simulink subsystem "VehicleSimulationRef"  (R2024b)
settings: Solver=VariableStepAuto  StartTime=0.0  StopTime=10.0  RelTol=1e-3
undefined symbols (not defined in the file): damp, flightTrajectory, Ka_accel, Kd_rate, Ki_angle, Kp_angle, omega, resetFlag, SimIn, SimPar, trajLen
libraries: starslibAxisTransformations x6, simulink_extras x5, dspstat3 x3, vrlib x3, aerolibanimutils x2, dspnetwork x1, aerolibfltsims x1, simulink x1
(part 2 of 2)

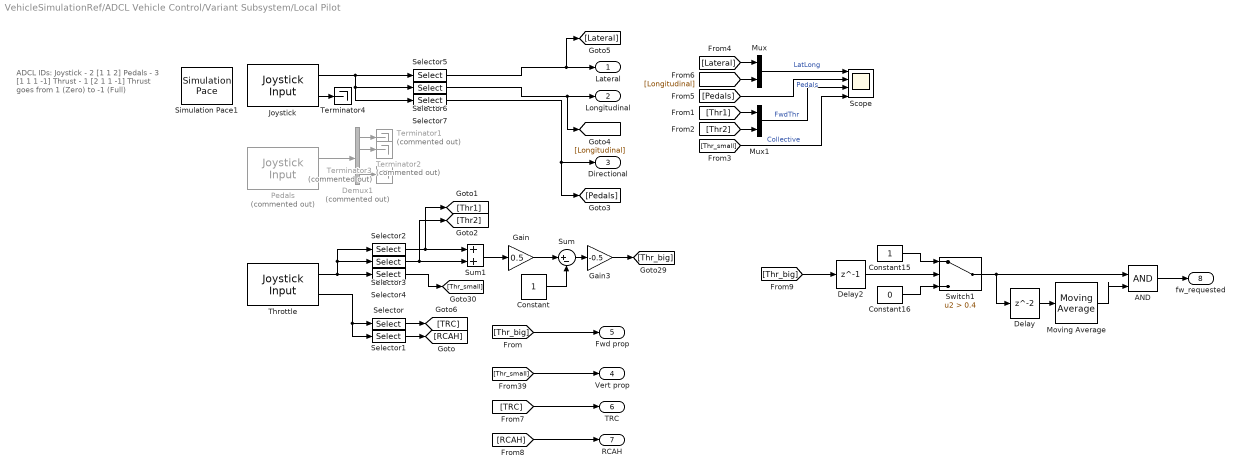
== system VehicleSimulationRef/ADCL Vehicle Control/Variant Subsystem/Local Pilot ==
  note: ADCL IDs:
      | Joystick - 2 [1 1 2]
      | Pedals - 3 [1 1 1 -1]
      | Thrust - 1 [2 1 1 -1]
      |
      | Thrust goes from 1 (Zero) to -1 (Full)
  AND : Logic  IconShape=distinctive  AllPortsSameDT=off  OutDataTypeStr=boolean
  Constant : Constant
  Constant15 : Constant
  Constant16 : Constant  Value=0
  Delay : Delay  InputProcessing=Columns as channels (frame based)  SampleTime=SimIn.Environment.Turbulence.dT
  Delay2 : Delay  DelayLength=1
  Demux1 : Demux  Commented=on  Outputs=[1 1 1 -1]
  Gain : Gain  Gain=0.5
  Gain3 : Gain  Gain=-0.5
  Joystick : vrlib/Joystick Input  joyid=2  adjustports=on  forcefeed=off
  Moving Average : dspstat3/Moving Average  Method=Sliding window  ForgettingFactorPort=off  SpecifyWindowLength=on  WindowLength=50  OverlapLength=49  AllowArbitraryInputLength=off  ForgettingFactor=0.9  SimulateUsing=Interpreted execution
  Mux : Mux  Inputs=2
  Mux1 : Mux  Inputs=2
  Pedals : vrlib/Joystick Input  Commented=on  joyid=3  adjustports=off  forcefeed=off
  Scope : Scope  NumInputPorts=4
  Selector : Selector  InputPortWidth=32  IndexOptions=Index vector (dialog)  Indices=24  OutputSizes=1
  Selector1 : Selector  InputPortWidth=32  IndexOptions=Index vector (dialog)  Indices=25  OutputSizes=1
  Selector2 : Selector  InputPortWidth=7  IndexOptions=Index vector (dialog)  Indices=3  OutputSizes=1
  Selector3 : Selector  InputPortWidth=7  IndexOptions=Index vector (dialog)  Indices=4  OutputSizes=1
  Selector4 : Selector  InputPortWidth=7  IndexOptions=Index vector (dialog)  Indices=5  OutputSizes=1
  Selector5 : Selector  InputPortWidth=4  IndexOptions=Index vector (dialog)  Indices=1  OutputSizes=1
  Selector6 : Selector  InputPortWidth=4  IndexOptions=Index vector (dialog)  Indices=2  OutputSizes=1
  Selector7 : Selector  InputPortWidth=4  IndexOptions=Index vector (dialog)  Indices=3  OutputSizes=1
  Simulation Pace1 : aerolibanimutils/Simulation Pace  SimulationPace=1  SleepMode=Auto  OutputPaceError=off  SampleTime=SimIn.Environment.Turbulence.dT
  Sum : Sum  Inputs=|+-
  Sum1 : Sum
  Switch1 : Switch  Criteria=u2 > Threshold  Threshold=0.4  SaturateOnIntegerOverflow=off  InputSameDT=off
  Terminator1 : Terminator  Commented=on
  Terminator2 : Terminator  Commented=on
  Terminator3 : Terminator  Commented=on
  Terminator4 : Terminator
  Throttle : vrlib/Joystick Input  joyid=1  adjustports=on  forcefeed=off
  Lateral : Outport
  Longitudinal : Outport  Port=2
  Directional : Outport  Port=3
  Vert prop : Outport  Port=4
  Fwd prop : Outport  Port=5
  TRC : Outport  Port=6
  RCAH : Outport  Port=7
  fw_requested : Outport  Port=8
  wires:
  [Thr_big] -> Delay2/1
  Constant16/1 -> Switch1/3
  Delay2/1 -> Switch1/2
  AND/1 -> fw_requested/1
  Constant15/1 -> Switch1/1
  Moving Average/1 -> AND/2
  Switch1/1 -> AND/1, Delay/1
  Delay/1 -> Moving Average/1
  Selector6/1 -> Longitudinal/1, [Longitudinal]
  Selector5/1 -> Lateral/1, [Lateral]
  Joystick/1 -> Selector5/1, Selector6/1, Selector7/1
  Selector1/1 -> [RCAH]
  [RCAH] -> RCAH/1
  [Thr_small] -> Vert prop/1
  [TRC] -> TRC/1
  Selector/1 -> [TRC]
  Throttle/2 -> Selector/1, Selector1/1
  [Thr_small] -> Scope/4  "Collective"
  Mux1/1 -> Scope/3  "FwdThr"
  [Pedals] -> Scope/2  "Pedals"
  Mux/1 -> Scope/1  "LatLong"
  [Thr2] -> Mux1/2
  [Thr1] -> Mux1/1
  [Lateral] -> Mux/1
  [Longitudinal] -> Mux/2
  Selector7/1 -> Directional/1, [Pedals]
  [Thr_big] -> Fwd prop/1
  Demux1/1 -> Terminator1/1
  Demux1/2 -> Terminator2/1
  Demux1/4 -> Terminator3/1
  Pedals/1 -> Demux1/1
  Gain3/1 -> [Thr_big]
  Constant/1 -> Sum/2
  Sum/1 -> Gain3/1
  Throttle/1 -> Selector4/1, Selector3/1, Selector2/1
  Sum1/1 -> Gain/1
  Selector2/1 -> [Thr1], Sum1/1
  Gain/1 -> Sum/1
  Selector3/1 -> [Thr2], Sum1/2
  Selector4/1 -> [Thr_small]
  Joystick/2 -> Terminator4/1

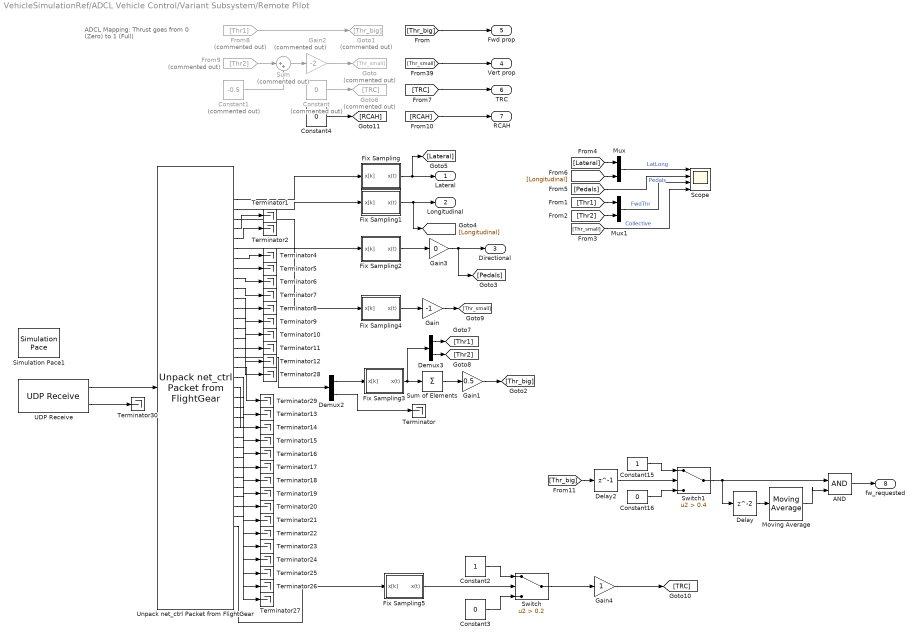
== system VehicleSimulationRef/ADCL Vehicle Control/Variant Subsystem/Remote Pilot ==
  note: ADCL Mapping:
      |
      | Thrust goes from 0 (Zero) to 1 (Full)
  AND : Logic  IconShape=distinctive  AllPortsSameDT=off  OutDataTypeStr=boolean
  Constant : Constant  Commented=on  Value=0
  Constant1 : Constant  Commented=on  Value=-0.5
  Constant15 : Constant
  Constant16 : Constant  Value=0
  Constant2 : Constant
  Constant3 : Constant  Value=0
  Constant4 : Constant  Value=0
  Delay : Delay  InputProcessing=Columns as channels (frame based)  SampleTime=SimIn.Environment.Turbulence.dT
  Delay2 : Delay  DelayLength=1
  Demux2 : Demux  Outputs=[2 2]
  Demux3 : Demux  Outputs=2
  Fix Sampling : Subsystem
  Fix Sampling1 : Subsystem
  Fix Sampling2 : Subsystem
  Fix Sampling3 : Subsystem
  Fix Sampling4 : Subsystem
  Fix Sampling5 : Subsystem
  From8 : From  Commented=on  GotoTag=Thr1
  From9 : From  Commented=on  GotoTag=Thr2
  Gain : Gain  Gain=-1
  Gain1 : Gain  Gain=0.5
  Gain2 : Gain  Commented=on  Gain=-2
  Gain3 : Gain  Gain=0
  Gain4 : Gain
  Goto : Goto  Commented=on  GotoTag=Thr_small
  Goto1 : Goto  Commented=on  GotoTag=Thr_big
  Goto6 : Goto  Commented=on  GotoTag=TRC
  Moving Average : dspstat3/Moving Average  Method=Sliding window  ForgettingFactorPort=off  SpecifyWindowLength=on  WindowLength=50  OverlapLength=49  AllowArbitraryInputLength=off  ForgettingFactor=0.9  SimulateUsing=Interpreted execution
  Mux : Mux  Inputs=2
  Mux1 : Mux  Inputs=2
  Scope : Scope  NumInputPorts=4
  Simulation Pace1 : aerolibanimutils/Simulation Pace  SimulationPace=1  SleepMode=Auto  OutputPaceError=off  SampleTime=SimIn.Environment.Turbulence.dT
  Sum : Sum  Commented=on  Inputs=|++
  Sum of Elements : Sum  Inputs=+
  Switch : Switch  Criteria=u2 > Threshold  Threshold=0.2  SaturateOnIntegerOverflow=off  InputSameDT=off
  Switch1 : Switch  Criteria=u2 > Threshold  Threshold=0.4  SaturateOnIntegerOverflow=off  InputSameDT=off
  Terminator{,1..2,4..30} (30 alike) : Terminator
  UDP Receive : dspnetwork/UDP Receive  localURL='0.0.0.0'  localPort=SimIn.simPortOutput  remoteURL=SimIn.simAddress  remotePort=-1  recvBufferSize=8192  dims=744  signalDatatype=uint8  isComplex=off  isVarSize=off  showBlockingTime=off  blockingTime=0  sampletime=-1  blockPlatform=[]
      settings: LibrarySourceBlock=dspsrcs4/UDP Receive
  Unpack net_ctrl Packet from FlightGear : aerolibfltsims/Unpack net_ctrl Packet from FlightGear  FlightGearVersion=v2019.1  ShowControlSurfacePositionOutputs=on  ShowEngineFuelOutputs=on  ShowLandingGearOutputs=on  ShowAvionicOutputs=off  ShowEnvironmentOutputs=off  SampleTime=-1  packetVersion=27
  Lateral : Outport
  Longitudinal : Outport  Port=2
  Directional : Outport  Port=3
  Vert prop : Outport  Port=4
  Fwd prop : Outport  Port=5
  TRC : Outport  Port=6
  RCAH : Outport  Port=7
  fw_requested : Outport  Port=8
  wires:
  Delay2/1 -> Switch1/2
  Constant16/1 -> Switch1/3
  Moving Average/1 -> AND/2
  Constant15/1 -> Switch1/1
  Switch1/1 -> AND/1, Delay/1
  [Thr_big] -> Delay2/1
  Delay/1 -> Moving Average/1
  AND/1 -> fw_requested/1
  Gain4/1 -> [TRC]
  Constant4/1 -> [RCAH]
  [RCAH] -> RCAH/1
  [TRC] -> TRC/1
  Switch/1 -> Gain4/1
  Constant3/1 -> Switch/3
  Constant2/1 -> Switch/1
  Unpack net_ctrl Packet from FlightGear/34 -> Fix Sampling5/1(x[k])
  Fix Sampling5/1(x(t)) -> Switch/2
  Gain3/1 -> [Pedals], Directional/1
  Gain/1 -> [Thr_small]
  Unpack net_ctrl Packet from FlightGear/6 -> Fix Sampling4/1(x[k])
  Fix Sampling4/1(x(t)) -> Gain/1
  Gain2/1 -> Goto/1
  Sum/1 -> Gain2/1
  From9/1 -> Sum/1
  Constant1/1 -> Sum/2
  From8/1 -> Goto1/1
  Fix Sampling3/1(x(t)) -> Sum of Elements/1, Demux3/1
  Fix Sampling2/1(x(t)) -> Gain3/1
  Fix Sampling1/1(x(t)) -> [Longitudinal], Longitudinal/1
  Fix Sampling/1(x(t)) -> [Lateral], Lateral/1
  UDP Receive/1 -> Unpack net_ctrl Packet from FlightGear/1
  UDP Receive/2 -> Terminator30/1
  Unpack net_ctrl Packet from FlightGear/18 -> Terminator29/1
  Unpack net_ctrl Packet from FlightGear/16 -> Terminator28/1
  Unpack net_ctrl Packet from FlightGear/33 -> Terminator27/1
  Unpack net_ctrl Packet from FlightGear/32 -> Terminator26/1
  Unpack net_ctrl Packet from FlightGear/31 -> Terminator25/1
  Unpack net_ctrl Packet from FlightGear/30 -> Terminator24/1
  Unpack net_ctrl Packet from FlightGear/29 -> Terminator23/1
  Unpack net_ctrl Packet from FlightGear/28 -> Terminator22/1
  Unpack net_ctrl Packet from FlightGear/27 -> Terminator21/1
  Unpack net_ctrl Packet from FlightGear/26 -> Terminator20/1
  Unpack net_ctrl Packet from FlightGear/25 -> Terminator19/1
  Unpack net_ctrl Packet from FlightGear/24 -> Terminator18/1
  Unpack net_ctrl Packet from FlightGear/23 -> Terminator17/1
  Unpack net_ctrl Packet from FlightGear/22 -> Terminator16/1
  Unpack net_ctrl Packet from FlightGear/21 -> Terminator15/1
  Unpack net_ctrl Packet from FlightGear/20 -> Terminator14/1
  Unpack net_ctrl Packet from FlightGear/19 -> Terminator13/1
  Unpack net_ctrl Packet from FlightGear/15 -> Terminator12/1
  Unpack net_ctrl Packet from FlightGear/14 -> Terminator11/1
  Unpack net_ctrl Packet from FlightGear/13 -> Terminator10/1
  Unpack net_ctrl Packet from FlightGear/12 -> Terminator9/1
  Unpack net_ctrl Packet from FlightGear/11 -> Terminator8/1
  Unpack net_ctrl Packet from FlightGear/10 -> Terminator7/1
  Unpack net_ctrl Packet from FlightGear/9 -> Terminator6/1
  Unpack net_ctrl Packet from FlightGear/8 -> Terminator5/1
  Unpack net_ctrl Packet from FlightGear/7 -> Terminator4/1
  Unpack net_ctrl Packet from FlightGear/5 -> Terminator2/1
  Unpack net_ctrl Packet from FlightGear/4 -> Terminator1/1
  Constant/1 -> Goto6/1
  Demux2/2 -> Terminator/1
  Gain1/1 -> [Thr_big]
  Demux3/2 -> [Thr2]
  Demux3/1 -> [Thr1]
  Unpack net_ctrl Packet from FlightGear/1 -> Fix Sampling/1(x[k])
  Unpack net_ctrl Packet from FlightGear/2 -> Fix Sampling1/1(x[k])
  [Thr_big] -> Fwd prop/1
  [Thr_small] -> Vert prop/1
  Unpack net_ctrl Packet from FlightGear/3 -> Fix Sampling2/1(x[k])
  [Longitudinal] -> Mux/2
  [Lateral] -> Mux/1
  [Thr1] -> Mux1/1
  [Thr2] -> Mux1/2
  Mux/1 -> Scope/1  "LatLong"
  [Pedals] -> Scope/2  "Pedals"
  Mux1/1 -> Scope/3  "FwdThr"
  [Thr_small] -> Scope/4  "Collective"
  Unpack net_ctrl Packet from FlightGear/17 -> Demux2/1
  Demux2/1 -> Fix Sampling3/1(x[k])
  Sum of Elements/1 -> Gain1/1

== system VehicleSimulationRef/ADCL Vehicle Control/Mapping To Output/Eng Dynamics Compensation/Default ==
  Eng_Des : Inport
  Eng_Cmd : Outport
  wires:
  Eng_Des/1 -> Eng_Cmd/1

== system VehicleSimulationRef/ADCL Vehicle Control/Mapping To Output/Eng Dynamics Compensation/First Order ==
  note: “Cancel” the lag from the First Order dynamics by commanding a value that anticipates the needed deflection rate. This formula “inverts” the first-order lag.
  Eng_Des : Inport
  Derivative : Derivative
  Sum : Sum  Inputs=|++
  tau : Gain  Gain=1 ./ (2 * pi * SimPar.Engine.BW)
  Eng_Cmd : Outport
  wires:
  tau/1 -> Sum/2
  Sum/1 -> Eng_Cmd/1
  Derivative/1 -> tau/1
  Eng_Des/1 -> Derivative/1, Sum/1

== system VehicleSimulationRef/ADCL Vehicle Control/Mapping To Output/Surf Dynamics Compensation/Default ==
  Surf_Des : Inport
  Surf_Cmd : Outport
  wires:
  Surf_Des/1 -> Surf_Cmd/1

== system VehicleSimulationRef/ADCL Vehicle Control/Mapping To Output/Surf Dynamics Compensation/First Order ==
  note: “Cancel” the lag from the First Order dynamics by commanding a value that anticipates the needed deflection rate. This formula “inverts” the first-order lag.
  Surf_Des : Inport
  Derivative : Derivative
  Sum : Sum  Inputs=|++
  tau : Gain  Gain=1 ./ (2 * pi * SimPar.Actuator.BW)
  Surf_Cmd : Outport
  wires:
  tau/1 -> Sum/2
  Surf_Des/1 -> Sum/1, Derivative/1
  Derivative/1 -> tau/1
  Sum/1 -> Surf_Cmd/1

== system VehicleSimulationRef/ADCL Vehicle Control/Pilot Command Filtering/Translational Rate Command (TRC)/Linear controller ==
  ref : Inport
  ref_dot : Inport  Port=2
  x_dot : Inport  Port=3
  notTRC : Inport  Port=4
  Gain : Gain  Gain=Kp
  Gain1 : Gain  Gain=Ki
  Gain2 : Gain  Gain=Ka
  Integrator : Integrator  ExternalReset=level
  Sum : Sum  Inputs=|+-
  Sum1 : Sum  Inputs=+++
  req : Outport
  wires:
  notTRC/1 -> Integrator/2
  Gain2/1 -> Sum1/1
  ref_dot/1 -> Gain2/1
  Integrator/1 -> Sum1/3
  Gain/1 -> Sum1/2
  Sum1/1 -> req/1
  Gain1/1 -> Integrator/1
  Sum/1 -> Gain/1, Gain1/1
  x_dot/1 -> Sum/2
  ref/1 -> Sum/1

== system VehicleSimulationRef/ADCL Vehicle Control/Pilot Command Filtering/Translational Rate Command (TRC)/Reference model ==
  xy_dot_comm : Inport
  notTRC : Inport  Port=2
  xy_dot_0 : Inport  Port=3
  1/Tv : Gain  Gain=1/Tv
  Constant1 : Constant  Value=0
  Integrator : Integrator  ExternalReset=level  InitialConditionSource=external
  Sum : Sum  Inputs=|+-
  Switch : Switch  Criteria=u2 ~= 0  SaturateOnIntegerOverflow=off  InputSameDT=off
  ref : Outport
  ref_dot : Outport  Port=2
  wires:
  1/Tv/1 -> Switch/3
  Constant1/1 -> Switch/1
  xy_dot_0/1 -> Integrator/3
  notTRC/1 -> Integrator/2, Switch/2
  Sum/1 -> 1/Tv/1
  xy_dot_comm/1 -> Sum/1
  Switch/1 -> Integrator/1, ref_dot/1
  Integrator/1 -> Sum/2, ref/1

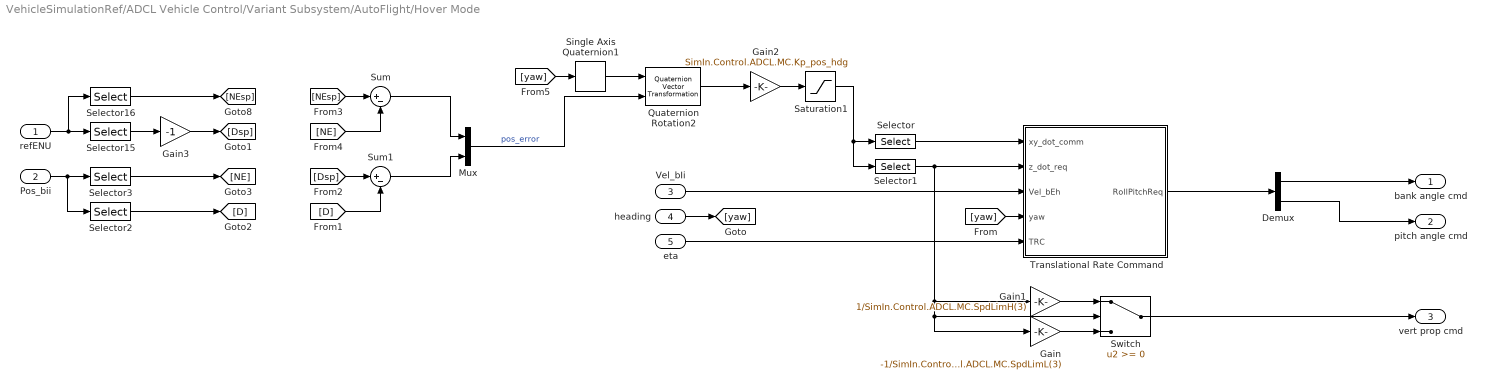
== system VehicleSimulationRef/ADCL Vehicle Control/Variant Subsystem/AutoFlight/Hover Mode ==
  refENU : Inport
  Pos_bii : Inport  Port=2
  Vel_bIi : Inport  Port=3
  heading : Inport  Port=4
  eta : Inport  Port=5
  Demux : Demux  Outputs=2
  Gain : Gain  Gain=-1/SimIn.Control.ADCL.MC.SpdLimL(3)
  Gain1 : Gain  Gain=1/SimIn.Control.ADCL.MC.SpdLimH(3)
  Gain2 : Gain  Gain=SimIn.Control.ADCL.MC.Kp_pos_hdg
  Gain3 : Gain  Gain=-1
  Mux : Mux  Inputs=2
  Quaternion Rotation2 : starslibAxisTransformations/Quaternion Vector Transformation  n=0
  Saturation1 : Saturate  UpperLimit=SimIn.Control.ADCL.MC.SpdLimH  LowerLimit=SimIn.Control.ADCL.MC.SpdLimL
  Selector : Selector  InputPortWidth=3  IndexOptions=Index vector (dialog)  Indices=[1 2]  OutputSizes=1
  Selector1 : Selector  InputPortWidth=3  IndexOptions=Index vector (dialog)  Indices=3  OutputSizes=1
  Selector15 : Selector  InputPortWidth=3  IndexOptions=Index vector (dialog)  Indices=3  OutputSizes=1
  Selector16 : Selector  InputPortWidth=3  IndexOptions=Index vector (dialog)  Indices=[2 1]  OutputSizes=1
  Selector2 : Selector  InputPortWidth=3  IndexOptions=Index vector (dialog)  Indices=3  OutputSizes=1
  Selector3 : Selector  InputPortWidth=3  IndexOptions=Index vector (dialog)  Indices=[1 2]  OutputSizes=1
  Single Axis Quaternion1 : starslibAxisTransformations/Single Axis Quaternion  RotAxis=z  n=0
  Sum : Sum  Inputs=|+-
  Sum1 : Sum  Inputs=|+-
  Switch : Switch  SaturateOnIntegerOverflow=off  InputSameDT=off
  Translational Rate Command : Subsystem
  bank angle cmd : Outport
  pitch angle cmd : Outport  Port=2
  vert prop cmd : Outport  Port=3
  wires:
  refENU/1 -> Selector16/1, Selector15/1
  Pos_bii/1 -> Selector2/1, Selector3/1
  Selector15/1 -> Gain3/1
  Selector16/1 -> [NEsp]
  Gain3/1 -> [Dsp]
  Selector3/1 -> [NE]
  Selector2/1 -> [D]
  Sum/1 -> Mux/1
  Sum1/1 -> Mux/2
  [D] -> Sum1/2
  [Dsp] -> Sum1/1
  [NEsp] -> Sum/1
  [NE] -> Sum/2
  Mux/1 -> Quaternion Rotation2/2  "pos_error"
  Saturation1/1 -> Selector/1, Selector1/1
  Gain2/1 -> Saturation1/1
  Quaternion Rotation2/1 -> Gain2/1
  Selector1/1 -> Translational Rate Command/2(z_dot_req), Switch/2, Gain/1, Gain1/1
  Selector/1 -> Translational Rate Command/1(xy_dot_comm)
  [yaw] -> Translational Rate Command/4(yaw)
  Single Axis Quaternion1/1 -> Quaternion Rotation2/1
  [yaw] -> Single Axis Quaternion1/1
  Gain1/1 -> Switch/1
  Gain/1 -> Switch/3
  heading/1 -> [yaw]
  Demux/2 -> pitch angle cmd/1
  Vel_bIi/1 -> Translational Rate Command/3(Vel_bEh)
  Translational Rate Command/1(RollPitchReq) -> Demux/1
  Switch/1 -> vert prop cmd/1
  eta/1 -> Translational Rate Command/5(TRC)
  Demux/1 -> bank angle cmd/1

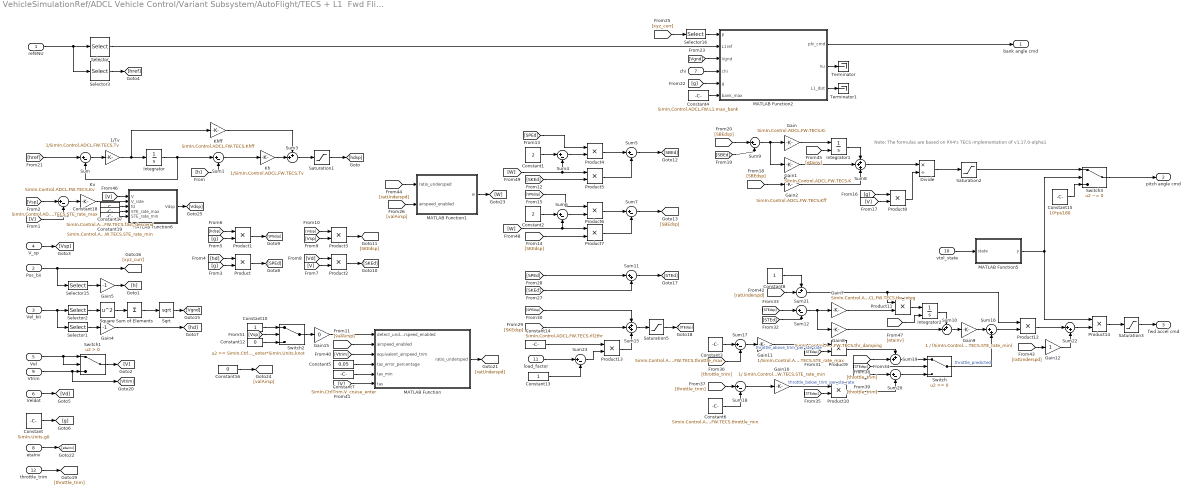
== system VehicleSimulationRef/ADCL Vehicle Control/Variant Subsystem/AutoFlight/TECS + L1  Fwd Flight ==
  note: Note: The formulas are based on PX4's TECS implementation of v1.17.0-alpha1
  refENU : Inport
  Pos_bii : Inport  Port=2
  Vel_bIi : Inport  Port=3
  V_sp : Inport  Port=4
  Vel : Inport  Port=5
  Veldot : Inport  Port=6
  chi : Inport  Port=7
  etaInv : Inport  Port=8
  Vtrim : Inport  Port=9
  vtol_state : Inport  Port=10
  load_factor : Inport  Port=11
  throttle_trim : Inport  Port=12
  1/Tv : Gain  Gain=1/SimIn.Control.ADCL.FW.TECS.Tv
  Constant : Constant  Value=SimIn.Units.g0
  Constant1 : Constant  Value=2
  Constant10 : Constant
  Constant12 : Constant  Value=0
  Constant13 : Constant
  Constant14 : Constant  Value=SimIn.Control.ADCL.FW.TECS.rll2thr
  Constant15 : Constant  Value=10*pi/180
  Constant16 : Constant  Value=0
  Constant17 : Constant  Value=SimIn.Control.ADCL.FW.TECS.fast_descend
  Constant18 : Constant  Value=SimIn.Control.ADCL.FW.TECS.STE_rate_max
  Constant19 : Constant  Value=SimIn.Control.ADCL.FW.TECS.STE_rate_min
  Constant2 : Constant  Value=2
  Constant3 : Constant  Value=SimIn.Control.ADCL.FW.TECS.throttle_max
  Constant4 : Constant  Value=SimIn.Control.ADCL.FW.L1.max_bank
  Constant5 : Constant  Value=0.05
  Constant6 : Constant  Value=SimIn.Control.ADCL.FW.TECS.throttle_min
  Constant7 : Constant  Value=SimIn.CtrlTrim.V_cruise_enter
  Constant8 : Constant
  Divide : Product  Inputs=*/
  Gain : Gain  Gain=SimIn.Control.ADCL.FW.TECS.Ki
  Gain1 : Gain  Gain=SimIn.Control.ADCL.FW.TECS.K
  Gain10 : Gain  Gain=1/ SimIn.Control.ADCL.FW.TECS.STE_rate_min
  Gain11 : Gain  Gain=1/SimIn.Control.ADCL.FW.TECS.STE_rate_max
  Gain12 : Gain
  Gain15 : Gain  Gain=0
  Gain2 : Gain  Gain=SimIn.Control.ADCL.FW.TECS.Kff
  Gain4 : Gain  Gain=-1
  Gain5 : Gain  Gain=-1
  Gain7 : Gain  Gain=SimIn.Control.ADCL.FW.TECS.thr_integ
  Gain8 : Gain  Gain=SimIn.Control.ADCL.FW.TECS.thr_damping
  Gain9 : Gain  Gain=1 / (SimIn.Control.ADCL.FW.TECS.STE_rate_max - SimIn.Control.ADCL.FW.TECS.STE_rate_min)
  Integrator : Integrator  InitialCondition=-SimIn.EOM.Pos_bii(3)
  Integrator1 : Integrator  ExternalReset=rising
  Integrator2 : Integrator  ExternalReset=rising
  Kh : Gain  Gain=1/SimIn.Control.ADCL.FW.TECS.Tv
  Khff : Gain  Gain=SimIn.Control.ADCL.FW.TECS.Khff
  Kv : Gain  Gain=SimIn.Control.ADCL.FW.TECS.Kv
  MATLAB Function : MATLAB Function  TreatAsAtomicUnit=on
  MATLAB Function1 : MATLAB Function  TreatAsAtomicUnit=on
  MATLAB Function2 : MATLAB Function  TreatAsAtomicUnit=on
  MATLAB Function5 : MATLAB Function  TreatAsAtomicUnit=on
  MATLAB Function6 : MATLAB Function  TreatAsAtomicUnit=on
  Product{,1..14} (15 alike) : Product
  Saturation1 : Saturate  UpperLimit=SimIn.Control.ADCL.FW.TECS.climb_rate  LowerLimit=-SimIn.Control.ADCL.FW.TECS.max_sink_rate
  Saturation2 : Saturate  UpperLimit=SimIn.Control.ADCL.FW.TECS.max_pitch  LowerLimit=SimIn.Control.ADCL.FW.TECS.min_pitch
  Saturation3 : Saturate  UpperLimit=SimIn.Control.ADCL.FW.TECS.throttle_max  LowerLimit=SimIn.Control.ADCL.FW.TECS.throttle_min
  Saturation5 : Saturate  UpperLimit=SimIn.Control.ADCL.FW.TECS.STE_rate_max  LowerLimit=SimIn.Control.ADCL.FW.TECS.STE_rate_min
  Selector : Selector  InputPortWidth=3  IndexOptions=Index vector (dialog)  Indices=[2 1]  OutputSizes=1
  Selector1 : Selector  InputPortWidth=3  IndexOptions=Index vector (dialog)  Indices=3  OutputSizes=1
  Selector15 : Selector  InputPortWidth=3  IndexOptions=Index vector (dialog)  Indices=3  OutputSizes=1
  Selector16 : Selector  InputPortWidth=3  IndexOptions=Index vector (dialog)  Indices=[1 2]  OutputSizes=1
  Selector2 : Selector  InputPortWidth=3  IndexOptions=Index vector (dialog)  Indices=[1 2]  OutputSizes=1
  Selector3 : Selector  InputPortWidth=3  IndexOptions=Index vector (dialog)  Indices=3  OutputSizes=1
  Sqrt : Sqrt
  Square : Math  Operator=square
  Sum{,1..2,4..7,9,12,17..18,20,23} (13 alike) : Sum  Inputs=|+-
  Sum of Elements : Sum  Inputs=+
  Sum10 : Sum  Inputs=++|
  Sum11 : Sum  Inputs=|++
  Sum15 : Sum  Inputs=+++
  Sum16 : Sum  Inputs=|++
  Sum19 : Sum  Inputs=++|
  Sum21 : Sum  Inputs=+-|
  Sum22 : Sum  Inputs=|++
  Sum3 : Sum  Inputs=++|
  Sum8 : Sum  Inputs=+++
  Switch : Switch  SaturateOnIntegerOverflow=off  InputSameDT=off
  Switch1 : Switch  Criteria=u2 > Threshold  SaturateOnIntegerOverflow=off  InputSameDT=off
  Switch2 : Switch  Threshold=SimIn.CtrlTrim.V_cruise_enter*SimIn.Units.knot  SaturateOnIntegerOverflow=off  InputSameDT=off
  Switch3 : Switch  Criteria=u2 ~= 0  SaturateOnIntegerOverflow=off  InputSameDT=off
  Terminator : Terminator
  Terminator1 : Terminator
  bank angle cmd : Outport
  pitch angle cmd : Outport  Port=2
  fwd accel cmd : Outport  Port=3
  wires:
  Selector3/1 -> [href]
  Selector/1 -> MATLAB Function2/2(L1ref)
  refENU/1 -> Selector/1, Selector3/1
  MATLAB Function6/1(Vdsp) -> [Vdsp]
  Constant18/1 -> MATLAB Function6/4(STE_rate_max)
  Constant19/1 -> MATLAB Function6/5(STE_rate_min)
  Constant17/1 -> MATLAB Function6/3(fd)
  [V] -> MATLAB Function6/1(V)
  Constant16/1 -> [valAirsp]
  Selector16/1 -> MATLAB Function2/1(p)
  MATLAB Function5/1(y) -> Switch3/2, Product14/1
  throttle_trim/1 -> [throttle_trim]
  vtol_state/1 -> MATLAB Function5/1(state)
  Switch3/1 -> pitch angle cmd/1
  Product14/1 -> Saturation3/1
  Constant15/1 -> Switch3/3
  Product12/1 -> Sum22/1
  Sum16/1 -> Product12/2
  MATLAB Function2/1(phi_cmd) -> bank angle cmd/1
  Saturation2/1 -> Switch3/1
  Saturation3/1 -> fwd accel cmd/1
  Gain15/1 -> MATLAB Function/1(detect_underspeed_enabled)
  Saturation5/1 -> [STEdsp]
  Product13/1 -> Sum15/3
  Constant14/1 -> Product13/1
  Sum23/1 -> Product13/2
  Constant13/1 -> Sum23/2
  load_factor/1 -> Sum23/1
  [W] -> Product5/1, Sum4/2
  MATLAB Function1/1(w) -> [W]
  [etainv] -> Integrator2/2
  [Vsp] -> Switch2/2
  etaInv/1 -> [etainv]
  Switch2/1 -> Gain15/1
  Constant12/1 -> Switch2/3
  Constant10/1 -> Switch2/1
  [valAirsp] -> MATLAB Function/2(airspeed_enabled)
  [valAirsp] -> MATLAB Function1/2(airspeed_enabled)
  [ratUnderspd] -> MATLAB Function1/1(ratio_undersped)
  Gain12/1 -> Sum22/2
  Sum22/1 -> Product14/2
  [ratUnderspd] -> Gain12/1
  Gain8/1 -> Sum10/2
  Sum21/1 -> Product11/1, Product12/1
  Gain7/1 -> Product11/2
  Product11/1 -> Integrator2/1
  Sum10/1 -> Gain9/1
  [ratUnderspd] -> Sum21/2
  Constant8/1 -> Sum21/1
  MATLAB Function/1(ratio_undersped) -> [ratUnderspd]
  Constant7/1 -> MATLAB Function/5(tas_min)
  Constant5/1 -> MATLAB Function/4(tas_error_percentage)
  [V] -> MATLAB Function/6(tas)
  [Vtrim] -> MATLAB Function/3(equivalent_airspeed_trim)
  Vtrim/1 -> Switch1/3, [Vtrim]
  Vel/1 -> Switch1/1, Switch1/2
  Switch1/1 -> [V]
  Gain11/1 -> Product9/1  "throttle_above_trim_per_ste_rate"
  Gain10/1 -> Product10/1  "throttle_below_trim_per_ste_rate"
  Product10/1 -> Sum20/2
  [throttle_trim] -> Sum20/1
  Sum20/1 -> Switch/3
  Sum19/1 -> Switch/1
  [throttle_trim] -> Sum19/2
  [throttle_trim] -> Sum18/1
  [throttle_trim] -> Sum17/2
  Constant6/1 -> Sum18/2
  [STEdsp] -> Product10/2
  Sum18/1 -> Gain10/1
  Sum17/1 -> Gain11/1
  [STEdsp] -> Product9/2
  Constant3/1 -> Sum17/1
  Gain9/1 -> Sum16/1
  Switch/1 -> Sum16/2  "throttle_predicted"
  Product9/1 -> Sum19/1
  [STEdsp] -> Switch/2
  Integrator2/1 -> Sum10/1
  Sum12/1 -> Gain8/1, Gain7/1
  [STEdsp] -> Sum12/1
  [STEd] -> Sum12/2
  [SKEdsp] -> Sum15/2
  [SPEdsp] -> Sum15/1
  [SKEd] -> Sum11/2
  [SPEd] -> Sum11/1
  Sum15/1 -> Saturation5/1
  Sum11/1 -> [STEd]
  [etainv] -> Integrator1/2
  [xyz_curr] -> Selector16/1
  Pos_bii/1 -> Selector15/1, [xyz_curr]
  [Vgnd] -> MATLAB Function2/3(Vgnd)
  Gain5/1 -> [h]
  Selector15/1 -> Gain5/1
  Gain4/1 -> [hd]
  Selector1/1 -> Gain4/1
  [href] -> Sum/1
  MATLAB Function2/3(L1_dist) -> Terminator1/1
  MATLAB Function2/2(nu) -> Terminator/1
  Sqrt/1 -> [Vgnd]
  Square/1 -> Sum of Elements/1
  Sum of Elements/1 -> Sqrt/1
  Selector2/1 -> Square/1
  Vel_bIi/1 -> Selector1/1, Selector2/1
  Khff/1 -> Sum3/1
  Kh/1 -> Sum3/2
  Constant4/1 -> MATLAB Function2/6(bank_max)
  [g] -> MATLAB Function2/5(g)
  chi/1 -> MATLAB Function2/4(chi)
  [SBEd] -> Sum9/2
  [SBEdsp] -> Sum9/1
  Sum9/1 -> Gain/1, Gain1/1
  Sum8/1 -> Divide/1
  Gain2/1 -> Sum8/3
  [SBEdsp] -> Gain2/1
  Integrator1/1 -> Sum8/1
  Gain1/1 -> Sum8/2
  Gain/1 -> Integrator1/1
  Divide/1 -> Saturation2/1
  Product8/1 -> Divide/2
  [g] -> Product8/1
  [V] -> Product8/2
  Sum5/1 -> [SBEd]
  Sum7/1 -> [SBEdsp]
  Constant2/1 -> Sum6/1
  Sum6/1 -> Product6/2
  Product6/1 -> Sum7/1
  Product7/1 -> Sum7/2
  [SPEdsp] -> Product6/1
  [SKEdsp] -> Product7/2
  [SKEd] -> Product5/2
  [SPEd] -> Product4/1
  Product5/1 -> Sum5/2
  Product4/1 -> Sum5/1
  Sum4/1 -> Product4/2
  [W] -> Product7/1, Sum6/2
  Constant1/1 -> Sum4/1
  [Vd] -> Product2/1
  [V] -> Product2/2
  Product2/1 -> [SKEd]
  Product3/1 -> [SKEdsp]
  [Vsp] -> Product3/2
  [Vdsp] -> Product3/1
  [hdsp] -> Product1/1
  [g] -> Product1/2
  Product1/1 -> [SPEdsp]
  Product/1 -> [SPEd]
  [g] -> Product/2
  [hd] -> Product/1
  Constant/1 -> [g]
  Saturation1/1 -> [hdsp]
  [Vsp] -> Sum2/1
  Veldot/1 -> [Vd]
  [V] -> Sum2/2
  Kv/1 -> MATLAB Function6/2(V_rate)
  [h] -> Sum1/2
  Sum3/1 -> Saturation1/1
  Sum1/1 -> Kh/1
  Sum2/1 -> Kv/1
  V_sp/1 -> [Vsp]
  1/Tv/1 -> Integrator/1, Khff/1
  Sum/1 -> 1/Tv/1
  Integrator/1 -> Sum1/1, Sum/2

== system VehicleSimulationRef/ADCL Vehicle Control/Variant Subsystem/Remote Pilot/Fix Sampling ==
  note: This block keeps the signal from dropping to 0 when the UDP packets are missed or didn't arrive
  x[k] : Inport
  Memory : Memory
  Switch : Switch  Criteria=u2 ~= 0  SaturateOnIntegerOverflow=off  InputSameDT=off
  x(t) : Outport
  wires:
  x[k]/1 -> Switch/2, Switch/1
  Switch/1 -> Memory/1, x(t)/1
  Memory/1 -> Switch/3

== system VehicleSimulationRef/ADCL Vehicle Control/Variant Subsystem/Remote Pilot/Fix Sampling1 ==
  note: This block keeps the signal from dropping to 0 when the UDP packets are missed or didn't arrive
  x[k] : Inport
  Memory : Memory
  Switch : Switch  Criteria=u2 ~= 0  SaturateOnIntegerOverflow=off  InputSameDT=off
  x(t) : Outport
  wires:
  Memory/1 -> Switch/3
  Switch/1 -> x(t)/1, Memory/1
  x[k]/1 -> Switch/1, Switch/2

== system VehicleSimulationRef/ADCL Vehicle Control/Variant Subsystem/Remote Pilot/Fix Sampling2 ==
  note: This block keeps the signal from dropping to 0 when the UDP packets are missed or didn't arrive
  x[k] : Inport
  Memory : Memory
  Switch : Switch  Criteria=u2 ~= 0  SaturateOnIntegerOverflow=off  InputSameDT=off
  x(t) : Outport
  wires:
  x[k]/1 -> Switch/2, Switch/1
  Switch/1 -> Memory/1, x(t)/1
  Memory/1 -> Switch/3

== system VehicleSimulationRef/ADCL Vehicle Control/Variant Subsystem/Remote Pilot/Fix Sampling3 ==
  note: This block keeps the signal from dropping to 0 when the UDP packets are missed or didn't arrive
  x[k] : Inport
  Memory : Memory
  Switch : Switch  Criteria=u2 ~= 0  SaturateOnIntegerOverflow=off  InputSameDT=off
  x(t) : Outport
  wires:
  Memory/1 -> Switch/3
  Switch/1 -> x(t)/1, Memory/1
  x[k]/1 -> Switch/1, Switch/2

== system VehicleSimulationRef/ADCL Vehicle Control/Variant Subsystem/Remote Pilot/Fix Sampling4 ==
  note: This block keeps the signal from dropping to 0 when the UDP packets are missed or didn't arrive
  x[k] : Inport
  Memory : Memory
  Switch : Switch  Criteria=u2 ~= 0  SaturateOnIntegerOverflow=off  InputSameDT=off
  x(t) : Outport
  wires:
  x[k]/1 -> Switch/2, Switch/1
  Switch/1 -> Memory/1, x(t)/1
  Memory/1 -> Switch/3

== system VehicleSimulationRef/ADCL Vehicle Control/Variant Subsystem/Remote Pilot/Fix Sampling5 ==
  note: This block keeps the signal from dropping to 0 when the UDP packets are missed or didn't arrive
  x[k] : Inport
  Memory : Memory
  Switch : Switch  Criteria=u2 ~= 0  SaturateOnIntegerOverflow=off  InputSameDT=off
  x(t) : Outport
  wires:
  x[k]/1 -> Switch/2, Switch/1
  Switch/1 -> Memory/1, x(t)/1
  Memory/1 -> Switch/3

== system VehicleSimulationRef/ADCL Vehicle Control/Variant Subsystem/AutoFlight/Hover Mode/Translational Rate Command ==
  xy_dot_comm : Inport
  z_dot_req : Inport  Port=2
  Vel_bEh : Inport  Port=3
  yaw : Inport  Port=4
  TRC : Inport  Port=5
  Constant : Constant  Value=SimIn.Units.g0
  Constant1 : Constant  Value=0
  Constant3 : Constant  Value=0
  Linear controller : Subsystem  mask{Kp=[0.5; 0.5; 0.5], Ki=[0.25^2; 0.25^2; 0], Ka=[1; 1; 0]}
      mask prompts: Kp "Rate gain"; Ki "Rate integral gain"; Ka "Acceleration gain"
      mask DialogControl DescTextVar Prompt: Linear controllers of the two TRC channels
  MATLAB Function : MATLAB Function  TreatAsAtomicUnit=on
  Mux : Mux  Inputs=2
  Mux1 : Mux  Inputs=2
  NOT : Logic  Operator=NOT  IconShape=distinctive  AllPortsSameDT=off  OutDataTypeStr=boolean
  Quaternion Rotation2 : starslibAxisTransformations/Quaternion Vector Transformation  n=0
  Reference model : Subsystem  mask{Tv=3}
      mask prompts: Tv "Time constant"
      mask DialogControl DescTextVar Prompt: First order reference models for the two TRC channels
  Selector : Selector  InputPortWidth=3  IndexOptions=Index vector (dialog)  Indices=[1 2]  OutputSizes=1
  Single Axis Quaternion1 : starslibAxisTransformations/Single Axis Quaternion  RotAxis=z  n=0
  RollPitchReq : Outport
  wires:
  Constant3/1 -> MATLAB Function/2(yaw)
  Vel_bEh/1 -> Quaternion Rotation2/2
  Quaternion Rotation2/1 -> Selector/1, Linear controller/3(x_dot)
  Single Axis Quaternion1/1 -> Quaternion Rotation2/1
  [yaw] -> Single Axis Quaternion1/1
  xy_dot_comm/1 -> Reference model/1(xy_dot_comm)
  Selector/1 -> Reference model/3(xy_dot_0)
  [notTRC] -> Linear controller/4(notTRC)
  [notTRC] -> Reference model/2(notTRC)
  NOT/1 -> [notTRC]
  TRC/1 -> NOT/1
  [z_dot_req] -> Mux/2
  z_dot_req/1 -> [z_dot_req]
  yaw/1 -> [yaw]
  Constant1/1 -> Mux1/2
  Reference model/1(ref) -> Mux/1
  Mux1/1 -> Linear controller/2(ref_dot)
  Reference model/2(ref_dot) -> Mux1/1
  Mux/1 -> Linear controller/1(ref)
  Constant/1 -> MATLAB Function/3(g)
  Linear controller/1(req) -> MATLAB Function/1(xyz_req)
  MATLAB Function/1(RollPitchReq) -> RollPitchReq/1

== system VehicleSimulationRef/ADCL Vehicle Control/Variant Subsystem/AutoFlight/Hover Mode/Translational Rate Command/Linear controller ==
  ref : Inport
  ref_dot : Inport  Port=2
  x_dot : Inport  Port=3
  notTRC : Inport  Port=4
  Gain : Gain  Gain=Kp
  Gain1 : Gain  Gain=Ki
  Gain2 : Gain  Gain=Ka
  Integrator : Integrator  ExternalReset=level
  Sum : Sum  Inputs=|+-
  Sum1 : Sum  Inputs=+++
  req : Outport
  wires:
  notTRC/1 -> Integrator/2
  Gain2/1 -> Sum1/1
  ref_dot/1 -> Gain2/1
  Integrator/1 -> Sum1/3
  Gain/1 -> Sum1/2
  Sum1/1 -> req/1
  Gain1/1 -> Integrator/1
  Sum/1 -> Gain/1, Gain1/1
  x_dot/1 -> Sum/2
  ref/1 -> Sum/1

== system VehicleSimulationRef/ADCL Vehicle Control/Variant Subsystem/AutoFlight/Hover Mode/Translational Rate Command/Reference model ==
  xy_dot_comm : Inport
  notTRC : Inport  Port=2
  xy_dot_0 : Inport  Port=3
  1/Tv : Gain  Gain=1/Tv
  Constant1 : Constant  Value=0
  Integrator : Integrator  ExternalReset=level  InitialConditionSource=external  LimitOutput=on  UpperSaturationLimit=SimIn.Control.ADCL.MC.SpdLimH(1:2)  LowerSaturationLimit=SimIn.Control.ADCL.MC.SpdLimL(1:2)
  Sum : Sum  Inputs=|+-
  Switch : Switch  Criteria=u2 ~= 0  SaturateOnIntegerOverflow=off  InputSameDT=off
  ref : Outport
  ref_dot : Outport  Port=2
  wires:
  1/Tv/1 -> Switch/3
  Constant1/1 -> Switch/1
  xy_dot_0/1 -> Integrator/3
  notTRC/1 -> Integrator/2, Switch/2
  Sum/1 -> 1/Tv/1
  xy_dot_comm/1 -> Sum/1
  Switch/1 -> Integrator/1, ref_dot/1
  Integrator/1 -> Sum/2, ref/1

== matlab function VehicleSimulationRef/ADCL Vehicle Control/MATLAB Function3 ==
  data: euler input; rpyRates output; pqr input
function rpyRates = rpyRates(euler, pqr)
    rpyRates = euler_rates(euler, pqr);
end

== matlab function VehicleSimulationRef/ADCL Vehicle Control/Variant Subsystem/AutoFlight/Hover Mode/Translational Rate Command/MATLAB Function ==
  data: xyz_req input; RollPitchReq output; yaw input; g input
function RollPitchReq = trc_inversion(xyz_req, yaw, g)
    RollPitchReq = kinematic_inversion(xyz_req, yaw, g);
end

== stateflow chart VehicleSimulationRef/ADCL Vehicle Control/Chart1 ==
  state LANDING
    eta = 1;
  state HOVER
    eta = 1;
  state Init
  note: This chart manages blending between vertical-lift and forward-flight using the coefficient eta, with separate entry/exit speeds to provide hysteresis.
      | Hover: eta = 1
      | Transition_Fwd: eta decreases from 1 to 0 using an exp function (e.g. 30 - 90 kts)
      | Cruise: eta = 0
      | Transition_Fwd: eta increases from 0 to 1 using an exp function (e.g. 90 - 45kts)
  state TRANS_TO_MC
    eta_new = getBlendingCoeff(Vel,V_hover_enter,V_cruise_exit);
    eta = max(eta_prev, eta_new);
  state TRANS_TO_FW
    eta_new = getBlendingCoeff(Vel,V_hover_exit,V_cruise_enter);
    eta = min(eta_prev, eta_new);
  state CRUISE
    eta = 0;
  HOVER -> LANDING [order 2] : [TRC == 1]
  LANDING -> HOVER : [TRC == 0]
  (default) -> Init
  Init -> HOVER [order 2] : [Vel < V_hover_enter]
  Init -> CRUISE [order 1] : [Vel > V_cruise_enter]
  Init -> (junction 70) [order 3] : [Vel < V_cruise_exit]
  HOVER -> TRANS_TO_FW [order 1] : [fw_requested == 1 && duration (fw_requested == 1, sec) > 2]
  TRANS_TO_MC -> HOVER [order 1] : [(eta > 0.95 || Vel < V_hover_enter) && duration (fw_requested ==0, sec) > 2]
  (junction 70) -> TRANS_TO_FW [order 1] : [Vel > V_hover_exit]
  (junction 70) -> TRANS_TO_MC [order 2] : [Vel > V_hover_enter]
  TRANS_TO_MC -> TRANS_TO_FW [order 2] : [fw_requested == 1 && duration (fw_requested == 1, sec) > 2]
  TRANS_TO_FW -> TRANS_TO_MC [order 2] : [fw_requested == 0 && duration (fw_requested == 0, sec) > 2]
  TRANS_TO_FW -> CRUISE [order 1] : [(eta < 0.05 || Vel > V_cruise_enter) && duration (fw_requested == 1, sec) > 2]
  CRUISE -> TRANS_TO_MC : [fw_requested == 0  && duration (fw_requested ==0, sec) > 2]
  data: vel function_input; vel_hover function_input; vel_forward function_input; coeff function_output; fw_requested input; eta_prev input; Vel input; V_hover_exit input; V_hover_enter input; V_cruise_exit input; V_cruise_enter input; eta output; TRC input; eta_new local; vtol_state output Enum: vtol_stateModeType
  function coeff = getBlendingCoeff(vel,  vel_hover, vel_forward):
    | function coeff = getBlendingCoeff(vel,  vel_hover, vel_forward)
    |     coeff = blendingCoeff(vel,  vel_hover, vel_forward);
    | end

== matlab function VehicleSimulationRef/ADCL Vehicle Control/MATLAB Function6 ==
  settings: sampleTime=SimIn.Environment.Turbulence.dT
  data: G output; v output; FM_u input; uMin output size=[SimIn.numEngines+4,1]; I input; m input; reference input; observed input; euler input; eta input; limits input; u_curr input size=[SimIn.numEngines+4,1]; om_prop_bias input; alpha input; dt input; uMax output size=[SimIn.numEngines+4,1]; duMin output size=[SimIn.numEngines+4,1]; duMax output size=[SimIn.numEngines+4,1]; Wv output; Wu output; u_d output size=[SimIn.numEngines+4,1]; du_d output size=[SimIn.numEngines+4,1]
function [G, v, uMin, uMax, duMin, duMax, Wv, Wu, u_d, du_d] = setupWLS(FM_u, I, m, reference, observed, euler, eta, limits, u_curr, om_prop_bias, alpha, dt)
    [G, v, uMin, uMax, duMin, duMax, Wv, Wu, u_d, du_d] = INDI_control(FM_u, I, m, reference, observed, euler, eta, limits, u_curr, om_prop_bias, alpha, dt);
end

== matlab function VehicleSimulationRef/ADCL Vehicle Control/MATLAB Function4 ==
  data: u_curr input; u_limits output; PosLimits input; RateLimits input
function u_limits   = limitFlaperon(u_curr, PosLimits, RateLimits)
    u_limits   = limitFlap(u_curr, PosLimits, RateLimits);
end

== matlab function VehicleSimulationRef/ADCL Vehicle Control/Variant Subsystem/AutoFlight/TECS + L1  Fwd Flight/MATLAB Function ==
  data: detect_underspeed_enabled input; airspeed_enabled input; equivalent_airspeed_trim input; ratio_undersped output; tas_error_percentage input; tas_min input; tas input
function ratio_undersped = detectUnderspeed(detect_underspeed_enabled, airspeed_enabled, equivalent_airspeed_trim, tas_error_percentage, tas_min, tas)

if (~detect_underspeed_enabled || ~airspeed_enabled)
	ratio_undersped = 0.0;
	return;
end

tas_error_bound = tas_error_percentage * equivalent_airspeed_trim;
tas_underspeed_soft_bound = tas_error_percentage * equivalent_airspeed_trim;

tas_fully_undersped = max(tas_min - tas_error_bound - tas_underspeed_soft_bound, 0.0);
tas_starting_to_underspeed = max(tas_min - tas_error_bound, tas_fully_undersped);

den = max(tas_starting_to_underspeed - tas_fully_undersped, eps);
x = (tas - tas_fully_undersped) / den;
x = min(max(x, 0.0), 1.0);

ratio_undersped = 1.0 - x;
end

== matlab function VehicleSimulationRef/ADCL Vehicle Control/Variant Subsystem/AutoFlight/TECS + L1  Fwd Flight/MATLAB Function2 ==
  data: phi_cmd output; p input; L1ref input; nu output; Vgnd input; chi input; g input; bank_max input; L1_dist output
function [phi_cmd, nu, L1_dist] = L1_lateral_command(p, L1ref, Vgnd, chi, g, bank_max)
% L1_LATERAL_COMMAND  Compute lateral acceleration and bank command.

p = p(:).'; 
p = p(1:2);
L1ref = L1ref(:).'; 
L1ref = L1ref(1:2);

L1_vec = L1ref - p;
L1_dist = norm(L1_vec);

% Desired bearing to reference point (ground frame)
chi_ref = atan2(L1_vec(2), L1_vec(1));

% nu = wrap(chi_ref - chi) constrained to +/- 90deg
nu = wrapToPi(chi_ref - chi);
nu = max(min(nu, pi/2), -pi/2);

% L1 acceleration command
a_lat = (2 * Vgnd^2 / max(L1_dist, 1e-3)) * sin(nu);

% Convert to bank (coordinated turn)
phi_cmd = atan2(a_lat, g);

% Limit bank
phi_cmd = max(min(phi_cmd, bank_max), -bank_max);

end

== matlab function VehicleSimulationRef/ADCL Vehicle Control/Variant Subsystem/AutoFlight/TECS + L1  Fwd Flight/MATLAB Function1 ==
  data: ratio_undersped input; w output; airspeed_enabled input
function w = pitch_speed_weight(ratio_undersped, airspeed_enabled)
w = 1;
if (ratio_undersped > eps && airspeed_enabled)
	w = 2.0 * ratio_undersped + (1.0 - ratio_undersped) * w;
elseif (~airspeed_enabled)
	w = 0.0;
end

== matlab function VehicleSimulationRef/ADCL Vehicle Control/Variant Subsystem/AutoFlight/MATLAB Function ==
  data: phi input; n output
function n = load_factor(phi)
    n = 1 / max(cos(phi), eps);
end

== matlab function VehicleSimulationRef/ADCL Vehicle Control/Variant Subsystem/AutoFlight/TECS + L1  Fwd Flight/MATLAB Function6 ==
  data: V input; Vdsp output; V_rate input; fd input; STE_rate_max input; STE_rate_min input
function Vdsp = limit_tas_rate(V, V_rate, fd, STE_rate_max, STE_rate_min)
    scaling_factor = (fd * 0.5 + 0.5) / max(V, eps);

    % Upper and lower bounds
    max_tas_rate_sp = scaling_factor * STE_rate_max;
    min_tas_rate_sp = scaling_factor * STE_rate_min;

    Vdsp = max(min(V_rate, max_tas_rate_sp), min_tas_rate_sp);
end

== matlab function VehicleSimulationRef/ADCL Vehicle Control/Variant Subsystem/AutoFlight/TECS + L1  Fwd Flight/MATLAB Function5 ==
  data: state input; y output
function y = fcn(state)

switch state
    case {vtol_stateModeType.TRANS_TO_FW, vtol_stateModeType.CRUISE}
        y = 1;
    otherwise % HOVER
        y = 0;
end

== matlab function VehicleSimulationRef/ADCL Vehicle Control/Variant Subsystem/AutoFlight/MATLAB Function3 ==
  settings: updateMethod=DISCRETE
  data: ENU_WPT output; pNED input; wptsENU input; L1 input; flag2End output; reset input; trajLen input; sTol input
function [ENU_WPT, flag2End] = pathGuidanceReference(pNED, wptsENU, L1, reset, trajLen, sTol)

    persistent wpts z N A B AB L2 good seg_len S endPtNED zEnd k_last have_last W s_hat initialized

    if isempty(initialized) || reset
        % Slice the input waypoints based on trajLen
        % Assuming wptsENU is [N_max x 3]
        wpts_subset = wptsENU(1:trajLen, :);
        
        wpts = wpts_subset(:,1:2);
        z = wpts_subset(:,3);
        N = size(wpts,1);
        
        % Segment vectors and squared lengths
        A = wpts(1:end-1,:);
        B = wpts(2:end,:);
        AB = B - A;
        L2 = sum(AB.^2, 2);
        good = L2 > 1e-12;
        
        % Path distance (Stationing)
        seg_len = sqrt(L2);
        seg_len(~good) = 0;
        S = [0; cumsum(seg_len)];
        
        % Search window logic
        window_dist = 100; % ft
        valid_segs = seg_len(seg_len > 1e-6);
        if isempty(valid_segs)
            med_len = 1.0; 
        else
            med_len = median(valid_segs);
        end
        W = ceil(window_dist / med_len);
        W = min(max(W, 50), 1000);
        
        % End point for termination logic (NED)
        endPtNED = [ wpts_subset(end,2); wpts_subset(end,1); -wpts_subset(end,3) ];
        zEnd = z(end);
        
        % Reset tracking state
        have_last = false;
        k_last = 1;
        s_hat = 0; 
        initialized = true;
    end
    
    L1 = max(L1, 0);
    pENU = [pNED(2) pNED(1)];

    % Local window search around last best segment
    if have_last
        i0 = max(1, k_last - W);
        i1 = min(N-1, k_last + W);
        idx = (i0:i1).';
    else
        idx = (1:N-1).';
    end

    APi = pENU - A(idx,:);
    L2i = L2(idx);
    goodi = good(idx);
    ABi = AB(idx,:);

    u_i = zeros(size(L2i));
    u_i(goodi) = sum(APi(goodi,:) .* ABi(goodi,:), 2) ./ L2i(goodi);
    u_i = min(max(u_i,0),1);

    proj_i = A(idx,:) + ABi .* u_i;
    d2_i = sum((pENU - proj_i).^2,2);
    d2_i(~goodi) = inf;

    [d2min, local_k] = min(d2_i);
    k_best = idx(local_k);
    u_best = u_i(local_k);

    % Update persistents (YOU WERE MISSING THIS)
    k_last = k_best;
    have_last = true;

    % Global fallback if we are far away
    fallback_dist = 500; % ft (tune)
    if d2min > fallback_dist^2
        idx = (1:N-1).';

        APi = pENU - A(idx,:);
        L2i = L2(idx);
        goodi = good(idx);
        ABi = AB(idx,:);

        u_i = zeros(size(L2i));
        u_i(goodi) = sum(APi(goodi,:) .* ABi(goodi,:), 2) ./ L2i(goodi);
        u_i = min(max(u_i,0),1);

        proj_i = A(idx,:) + ABi .* u_i;
        d2_i = sum((pENU - proj_i).^2,2);
        d2_i(~goodi) = inf;

        [~, local_k] = min(d2_i);
        k_best = idx(local_k);
        u_best = u_i(local_k);

        k_last = k_best;
    end

    % Closest station
    S_closest = S(k_best) + u_best * seg_len(k_best);

     %%%%%%%%%%%%%%%%%%%%%%%%%%%%%%%%%%%%%%%%%%%%%%%%%%%%%%%%
    % If far away, snap (merge behavior)
    snap_dist = 50; % ft, tune
    if sqrt(d2min) > snap_dist
        s_hat = S_closest;
    else
        % Smoothly track closest station (prevents left/right chatter)
        alpha = 0.05;             % low-pass gain (tune)
        s_hat = (1-alpha)*s_hat + alpha*S_closest;
    
        % Also enforce monotonic progress if desired:
        s_hat = max(s_hat, S_closest - 10); % small allowance backwards
    end
     %%%%%%%%%%%%%%%%%%%%%%%%%%%%%%%%%%%%%%%%%%%%%%%%%%%%%%%%

    flag2End = norm(pNED(:) - endPtNED(:)) <= sTol;

    % Target station
    % S_target = S_closest + L1;
    S_target = s_hat + L1;

    if S_target >= S(end)
        L1refEN = wpts(end,:);
        % L1ref = [L1refEN(2) L1refEN(1)];
        altRef = zEnd;
        ENU_WPT = [L1refEN(1); L1refEN(2); altRef];
        return
    end

    % Find k_t with binary search
    lo = 1;
    hi = N;
    while hi - lo > 1
        mid = floor((lo + hi)/2);
        if S_target >= S(mid)
            lo = mid;
        else
            hi = mid;
        end
    end
    k_t = lo;

    % Interpolate
    Lk = seg_len(k_t);
    if Lk < 1e-12
        L1refEN = B(k_t,:);
        altRef = z(k_t+1);
    else
        u_t = (S_target - S(k_t)) / Lk;
        L1refEN = A(k_t,:) + u_t * AB(k_t,:);
        altRef = z(k_t) + u_t * (z(k_t+1) - z(k_t));
    end

    % L1ref = [L1refEN(2) L1refEN(1)];
    ENU_WPT = [L1refEN(1); L1refEN(2); altRef];
end

== matlab function VehicleSimulationRef/SimOut_Selection ==
  data: u input; SimOut output Bus: BUS_USER_SIM_OUT
function SimOut = fcn(u)

SimOut = mySimOutFunc(u);

== matlab function VehicleSimulationRef/ADCL Vehicle Control/Pilot Command Filtering/Translational Rate Command (TRC)/MATLAB Function ==
  data: xyz_req input; RollPitchReq output; yaw input; g input
function RollPitchReq = trc_inversion(xyz_req, yaw, g)
    RollPitchReq = kinematic_inversion(xyz_req, yaw, g);
end

== matlab function VehicleSimulationRef/ADCL Vehicle Control/MATLAB Function2 ==
  data: G input size=[5,SimIn.numEngines+4]; v input size=[5,1]; uMin input size=[SimIn.numEngines+4,1]; u output size=[SimIn.numEngines+4,1]; uMax input size=[SimIn.numEngines+4,1]; Wv input size=[5,5]; Wu input size=[SimIn.numEngines+4,SimIn.numEngines+4]; ud input size=[SimIn.numEngines+4,1]; W output size=[SimIn.numEngines+4,1]; iter output size=[1,1]
function [u, W, iter] = runWLS(G, v, uMin, uMax, Wv, Wu, ud)
    gam = 1e4;
    [u, W, iter] = activeSetWLS(G, v, uMin, uMax, Wv, Wu, ud, gam);
end
